simulink model "obsvIntegralSimul"  (R2016a)
settings: Solver=ode45  StartTime=0.0  StopTime=150  RelTol=1e-3
undefined symbols (not defined in the file or in its folder): A, B, C, F, G, Kd, Ki, L, Ts, x0, x_esht_0
settings Model: Creator=dimpa  LastModifiedBy=emil
settings DataIOCC: LimitDataPoints=on  SaveFormat=Array
settings DebuggingCC: SolverPrmCheckMsg=warning
settings HardwareCC: ProdBitPerPointer=32  ProdLargestAtomicFloat=None  ProdIntDivRoundTo=Undefined  ProdEndianess=Unspecified  ProdWordSize=32  ProdHWDeviceType=32-bit Generic
settings ModelReferenceCC: PropagateSignalLabelsOutOfModel=off
settings ConfigComp: CovModelRefEnable=Off  CovSFcnEnable=off

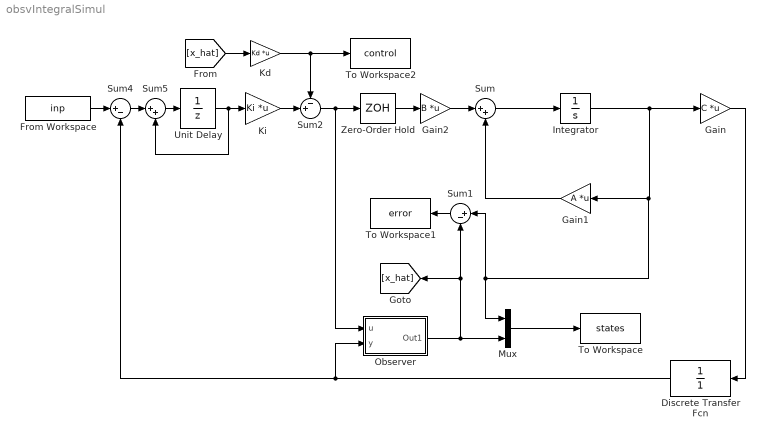
== system obsvIntegralSimul ==
  Discrete Transfer Fcn : DiscreteTransferFcn  Denominator=[1]  SampleTime=Ts
  From Workspace : FromWorkspace  VariableName=inp  SampleTime=0.1
  Gain : Gain  Gain=C  Multiplication=Matrix(K*u) (u vector)
  Gain1 : Gain  Gain=A  Multiplication=Matrix(K*u) (u vector)
  Gain2 : Gain  Gain=B  Multiplication=Matrix(K*u) (u vector)
  Integrator : Integrator  InitialCondition=x0
  Kd : Gain  Gain=Kd  Multiplication=Matrix(K*u) (u vector)
  Ki : Gain  Gain=Ki  Multiplication=Matrix(K*u) (u vector)
  Mux : Mux  Inputs=2
  Observer : Subsystem
  Sum : Sum  Inputs=|++
  Sum1 : Sum  Inputs=|+-
  Sum2 : Sum  Inputs=-+|
  Sum4 : Sum  Inputs=|+-  SaturateOnIntegerOverflow=on  InputSameDT=on  OutDataTypeStr=Inherit: Same as first input
  Sum5 : Sum  Inputs=|++  SaturateOnIntegerOverflow=on  InputSameDT=on  OutDataTypeStr=Inherit: Same as first input
  To Workspace : ToWorkspace  VariableName=states  SaveFormat=Structure With Time  SampleTime=-1
  To Workspace1 : ToWorkspace  VariableName=error  SaveFormat=Structure With Time  SampleTime=-1
  To Workspace2 : ToWorkspace  VariableName=control  SaveFormat=Structure With Time  SampleTime=-1
  Unit Delay : UnitDelay  SampleTime=Ts
  Zero-Order Hold : ZeroOrderHold  SampleTime=Ts
  wires:
  Gain2/1 -> Sum/1
  Sum/1 -> Integrator/1
  Gain1/1 -> Sum/2
  Gain/1 -> Discrete Transfer Fcn/1
  Sum2/1 -> Zero-Order Hold/1, Observer/1(u)
  Observer/1(Out1) -> Mux/2, [x_hat], Sum1/2
  Mux/1 -> To Workspace/1
  Discrete Transfer Fcn/1 -> Sum4/2, Observer/2(y)
  Sum1/1 -> To Workspace1/1
  Kd/1 -> Sum2/1, To Workspace2/1
  Zero-Order Hold/1 -> Gain2/1
  Ki/1 -> Sum2/2
  From Workspace/1 -> Sum4/1
  [x_hat] -> Kd/1
  Integrator/1 -> Mux/1, Sum1/1, Gain1/1, Gain/1
  Sum4/1 -> Sum5/1
  Sum5/1 -> Unit Delay/1
  Unit Delay/1 -> Sum5/2, Ki/1

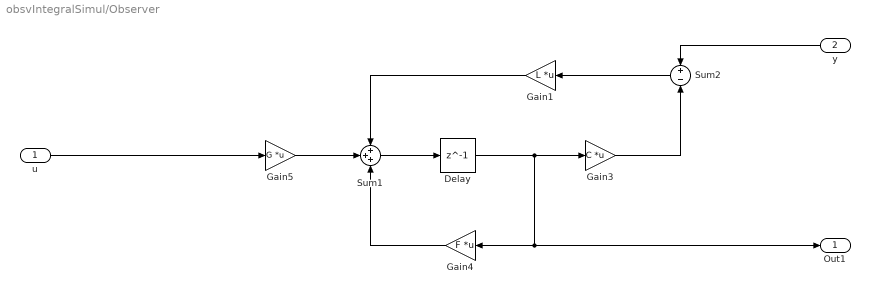
== system obsvIntegralSimul/Observer ==
  u : Inport
  y : Inport  Port=2
  Delay : Delay  DelayLength=1  InitialCondition=x_esht_0  SampleTime=0.1
  Gain1 : Gain  Gain=L  Multiplication=Matrix(K*u) (u vector)
  Gain3 : Gain  Gain=C  Multiplication=Matrix(K*u) (u vector)
  Gain4 : Gain  Gain=F  Multiplication=Matrix(K*u) (u vector)
  Gain5 : Gain  Gain=G  Multiplication=Matrix(K*u) (u vector)
  Sum1 : Sum  Inputs=+++
  Sum2 : Sum  Inputs=+-
  Out1 : Outport
  wires:
  Gain5/1 -> Sum1/2
  Sum1/1 -> Delay/1
  Delay/1 -> Gain3/1, Out1/1, Gain4/1
  Gain4/1 -> Sum1/3
  Gain3/1 -> Sum2/2
  u/1 -> Gain5/1
  y/1 -> Sum2/1
  Sum2/1 -> Gain1/1
  Gain1/1 -> Sum1/1
